simulink model "Lab2PartB1"  (R2023b)
settings: Solver=VariableStepAuto  StartTime=0.0  StopTime=10.0  RelTol=1e-3
settings Model: Creator=m96sz  LastModifiedBy=m96sz

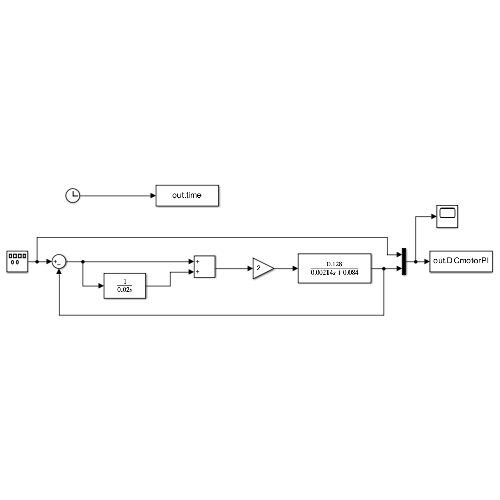
[thumbnail: Simulink's stored preview of the top-level diagram]
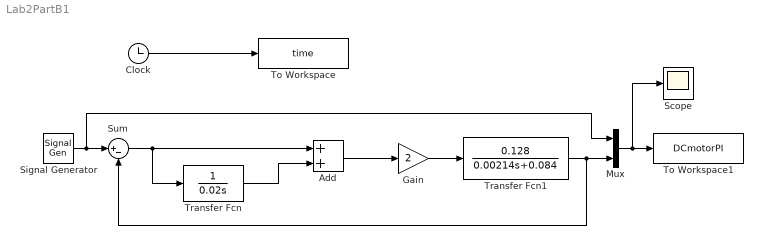
== system Lab2PartB1 ==
  Add : Sum
  Clock : Clock
  Gain : Gain  Gain=2
  Mux : Mux  Inputs=2
  Scope : Scope
  Signal Generator : SignalGenerator  Units=rad/sec
  Sum : Sum  Inputs=|+-
  To Workspace : ToWorkspace  VariableName=time  SaveFormat=Timeseries  SampleTime=-1
  To Workspace1 : ToWorkspace  VariableName=DCmotorPI  SaveFormat=Timeseries  SampleTime=-1
  Transfer Fcn : TransferFcn  Denominator=[0.02 0]
  Transfer Fcn1 : TransferFcn  Numerator=[0.128]  Denominator=[0.00214 0.084]
  wires:
  Clock/1 -> To Workspace/1
  Signal Generator/1 -> Mux/1, Sum/1
  Sum/1 -> Transfer Fcn/1, Add/1
  Transfer Fcn/1 -> Add/2
  Add/1 -> Gain/1
  Gain/1 -> Transfer Fcn1/1
  Transfer Fcn1/1 -> Sum/2, Mux/2
  Mux/1 -> Scope/1, To Workspace1/1
